simulink model "Baterie"  (R2023b)
settings: Solver=FixedStepAuto  StartTime=0.0  StopTime=10000  FixedStep=0.01  RelTol=1e-3
undefined symbols (not defined in the file): Cp_sys, Cp_sys1, Cp_sys2, Rp_sys, Rp_sys1, Rp_sys2, Rs_sys
libraries: simulink x1
settings Model: Creator=tudorn  LastModifiedBy=tudorn

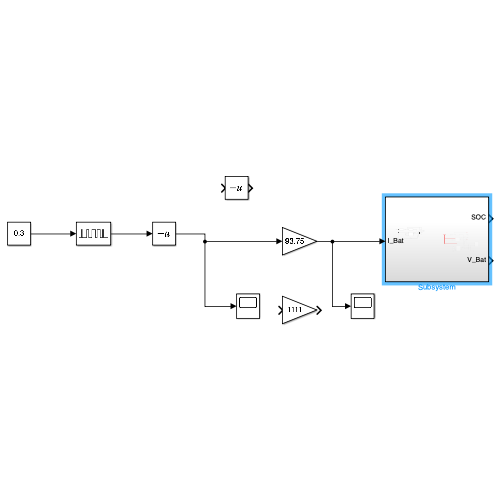
[thumbnail: Simulink's stored preview of the top-level diagram]
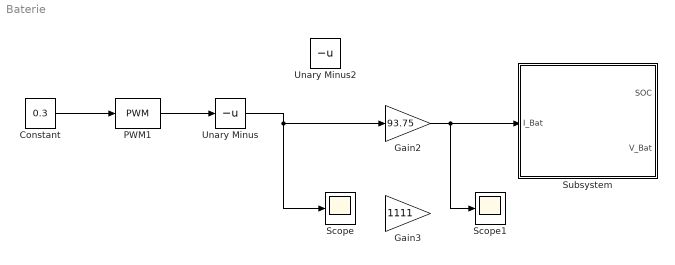
== system Baterie ==
  Constant : Constant  Value=0.3
  Gain2 : Gain  Gain=93.75
  Gain3 : Gain  Gain=1111
  PWM1 : simulink/Discontinuities/PWM  DisableCoverage=on  Period=1000  InitialDelay=0  DisallowZeroDutyCycle=off  RunAtFixedTimeIntervals=on  SampleTime=0.01
  Scope : Scope
  Scope1 : Scope
  Subsystem : Subsystem
  Unary Minus : UnaryMinus
  Unary Minus2 : UnaryMinus
  wires:
  Constant/1 -> PWM1/1
  Gain2/1 -> Scope1/1, Subsystem/1(I_Bat)
  PWM1/1 -> Unary Minus/1
  Unary Minus/1 -> Gain2/1, Scope/1

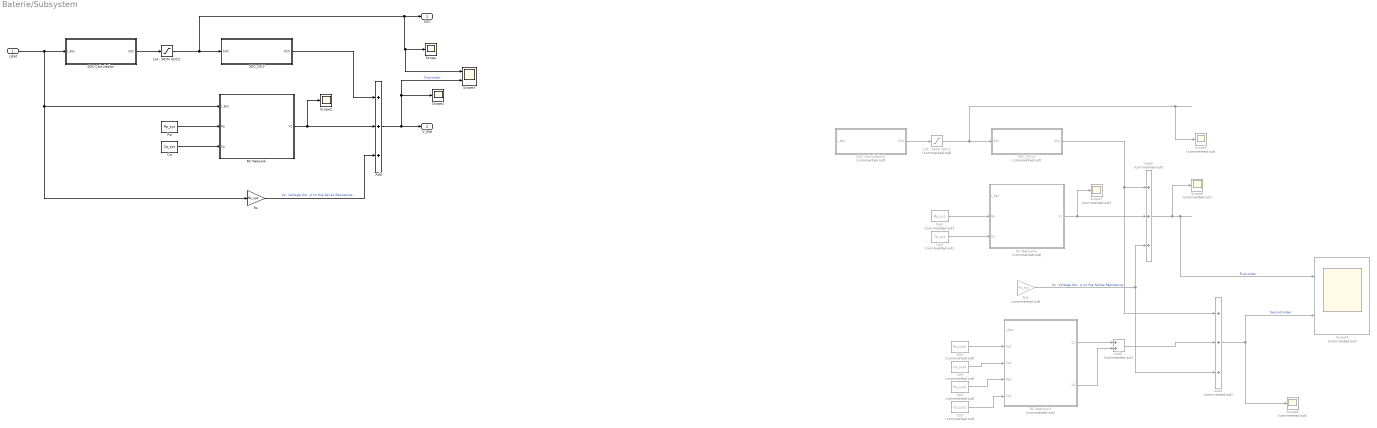
== system Baterie/Subsystem ==
  I_Bat : Inport
  (14 - 96)% SOC1 : Saturate  Commented=on  UpperLimit=96  LowerLimit=14
  (14 - 96)% SOC2 : Saturate  UpperLimit=96  LowerLimit=14
  Add : Sum  Inputs=+++
  Add3 : Sum  Commented=on  Inputs=+++
  Add4 : Sum  Commented=on  Inputs=+++
  Add5 : Sum  Commented=on
  Cp : Constant  Value=Cp_sys
  Cp3 : Constant  Commented=on  Value=Cp_sys
  Cp4 : Constant  Commented=on  Value=Cp_sys1
  Cp5 : Constant  Commented=on  Value=Cp_sys2
  RC Network : Subsystem
  RC Network2 : Subsystem  Commented=on
  RC Network3 : Subsystem  Commented=on
  Rp : Constant  Value=Rp_sys
  Rp3 : Constant  Commented=on  Value=Rp_sys
  Rp4 : Constant  Commented=on  Value=Rp_sys1
  Rp5 : Constant  Commented=on  Value=Rp_sys2
  Rs : Gain  Gain=Rs_sys
  Rs1 : Gain  Commented=on  Gain=Rs_sys
  SOC Calculation : Subsystem
  SOC Calculation1 : Subsystem  Commented=on
  SOC_OCV : Subsystem
  SOC_OCV1 : Subsystem  Commented=on
  Scope : Scope
  Scope1 : Scope
  Scope2 : Scope
  Scope3 : Scope  NumInputPorts=2
  Scope{5..8} (4 alike) : Scope  Commented=on
  Scope9 : Scope  Commented=on  NumInputPorts=2
  SOC : Outport
  V_Bat : Outport  Port=2
  wires:
  RC Network/1(V1) -> Scope2/1, Add/2
  SOC_OCV/1(OCV) -> Add/1
  Rp/1 -> RC Network/2(Rp)
  Cp/1 -> RC Network/3(Cp)
  I_Bat/1 -> SOC Calculation/1(I_Bat), Rs/1, RC Network/1(I_Bat)
  Add/1 -> Scope3/2, Scope1/1, V_Bat/1  "First-order"
  Rs/1 -> Add/3  "Vs - Voltage drop on the Series Resistance"
  Add4/1 -> Scope9/2, Scope8/1  "Second order"
  Add5/1 -> Add4/2
  RC Network3/2(V2) -> Add5/2
  RC Network3/1(V1) -> Add5/1
  Cp5/1 -> RC Network3/5(Cp2)
  Rp5/1 -> RC Network3/4(Rp2)
  Rp4/1 -> RC Network3/2(Rp1)
  Cp4/1 -> RC Network3/3(Cp1)
  (14 - 96)% SOC1/1 -> SOC_OCV1/1(SOC), Scope5/1
  Rs1/1 -> Add3/3, Add4/3  "Vs - Voltage drop on the Series Resistance"
  SOC Calculation1/1(SOC) -> (14 - 96)% SOC1/1
  Add3/1 -> Scope9/1, Scope6/1  "First-order"
  ? -> RC Network2/1(I_Bat), Rs1/1, RC Network3/1(I_Bat), SOC Calculation1/1(I_Bat)
  Cp3/1 -> RC Network2/3(Cp)
  Rp3/1 -> RC Network2/2(Rp)
  SOC_OCV1/1(OCV) -> Add3/1, Add4/1
  RC Network2/1(V1) -> Add3/2, Scope7/1
  SOC Calculation/1(SOC) -> (14 - 96)% SOC2/1
  (14 - 96)% SOC2/1 -> Scope3/1, Scope/1, SOC/1, SOC_OCV/1(SOC)

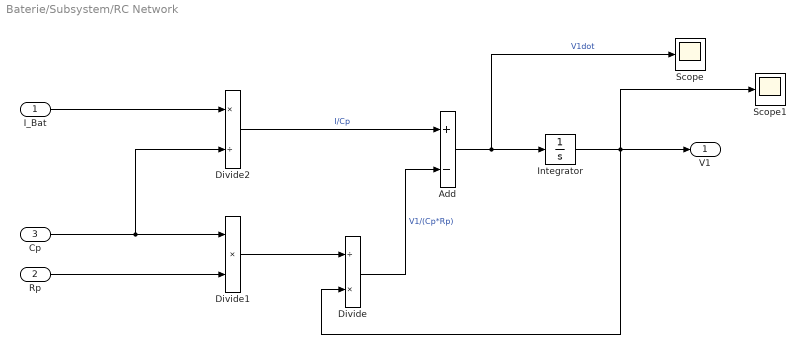
== system Baterie/Subsystem/RC Network ==
  I_Bat : Inport
  Rp : Inport  Port=2
  Cp : Inport  Port=3
  Add : Sum  Inputs=+-
  Divide : Product  Inputs=/*
  Divide1 : Product  Inputs=**
  Divide2 : Product  Inputs=*/
  Integrator : Integrator
  Scope : Scope
  Scope1 : Scope
  V1 : Outport
  wires:
  Cp/1 -> Divide2/2, Divide1/1
  Rp/1 -> Divide1/2
  I_Bat/1 -> Divide2/1
  Divide2/1 -> Add/1  "I/Cp"
  Add/1 -> Scope/1, Integrator/1  "V1dot"
  Divide/1 -> Add/2  "V1/(Cp*Rp)"
  Divide1/1 -> Divide/1
  Integrator/1 -> Scope1/1, V1/1, Divide/2

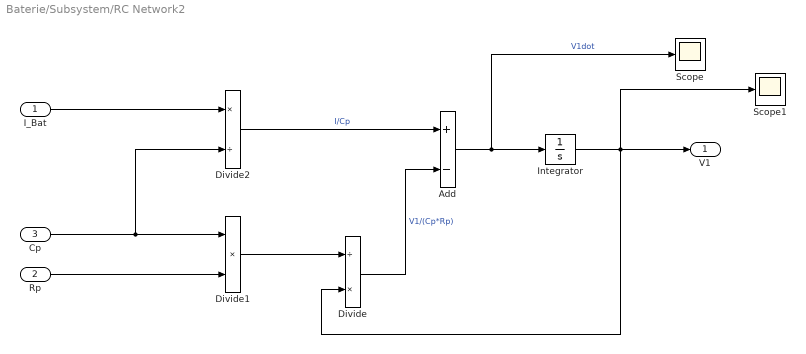
== system Baterie/Subsystem/RC Network2 ==
  I_Bat : Inport
  Rp : Inport  Port=2
  Cp : Inport  Port=3
  Add : Sum  Inputs=+-
  Divide : Product  Inputs=/*
  Divide1 : Product  Inputs=**
  Divide2 : Product  Inputs=*/
  Integrator : Integrator
  Scope : Scope
  Scope1 : Scope
  V1 : Outport
  wires:
  Integrator/1 -> Divide/2, V1/1, Scope1/1
  Divide1/1 -> Divide/1
  Divide/1 -> Add/2  "V1/(Cp*Rp)"
  Add/1 -> Integrator/1, Scope/1  "V1dot"
  Divide2/1 -> Add/1  "I/Cp"
  I_Bat/1 -> Divide2/1
  Rp/1 -> Divide1/2
  Cp/1 -> Divide1/1, Divide2/2

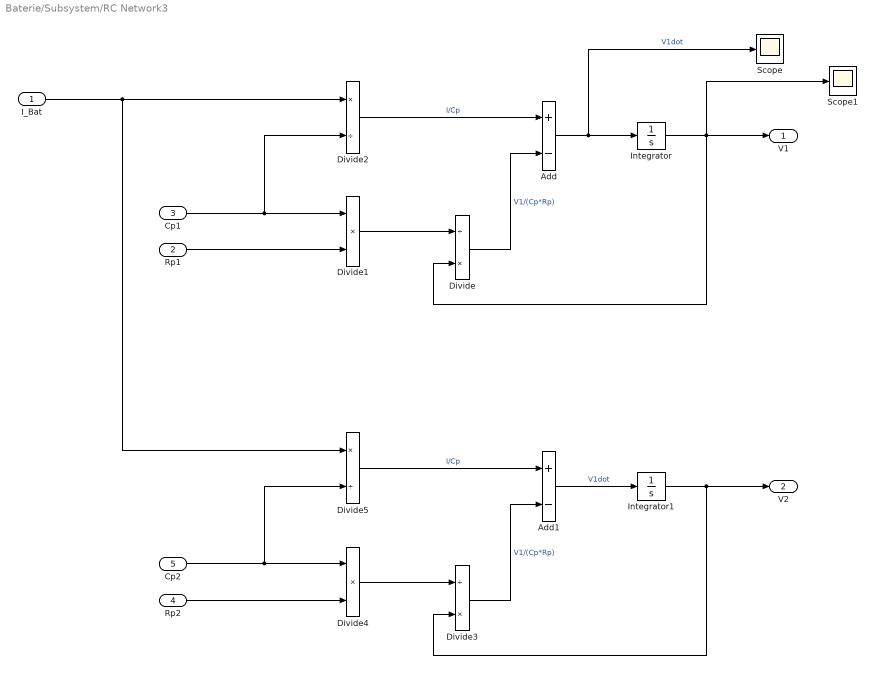
== system Baterie/Subsystem/RC Network3 ==
  I_Bat : Inport
  Rp1 : Inport  Port=2
  Cp1 : Inport  Port=3
  Rp2 : Inport  Port=4
  Cp2 : Inport  Port=5
  Add : Sum  Inputs=+-
  Add1 : Sum  Inputs=+-
  Divide : Product  Inputs=/*
  Divide1 : Product  Inputs=**
  Divide2 : Product  Inputs=*/
  Divide3 : Product  Inputs=/*
  Divide4 : Product  Inputs=**
  Divide5 : Product  Inputs=*/
  Integrator : Integrator
  Integrator1 : Integrator
  Scope : Scope
  Scope1 : Scope
  V1 : Outport
  V2 : Outport  Port=2
  wires:
  Divide5/1 -> Add1/1  "I/Cp"
  Rp2/1 -> Divide4/2
  Cp2/1 -> Divide4/1, Divide5/2
  Divide3/1 -> Add1/2  "V1/(Cp*Rp)"
  Divide4/1 -> Divide3/1
  Integrator1/1 -> Divide3/2, V2/1
  Add1/1 -> Integrator1/1  "V1dot"
  Integrator/1 -> Divide/2, V1/1, Scope1/1
  Divide1/1 -> Divide/1
  Divide/1 -> Add/2  "V1/(Cp*Rp)"
  Add/1 -> Integrator/1, Scope/1  "V1dot"
  Divide2/1 -> Add/1  "I/Cp"
  I_Bat/1 -> Divide2/1, Divide5/1
  Rp1/1 -> Divide1/2
  Cp1/1 -> Divide1/1, Divide2/2

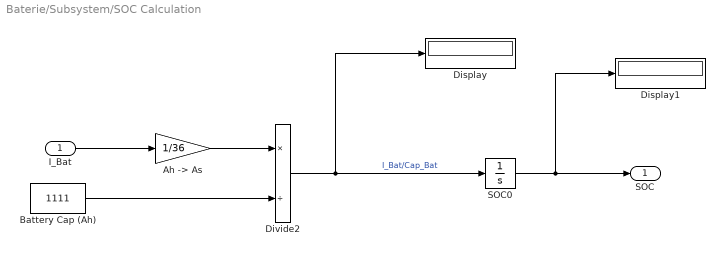
== system Baterie/Subsystem/SOC Calculation ==
  I_Bat : Inport
  "Ah -> As" : Gain  Gain=1/36
  Battery Cap (Ah) : Constant  Value=1111
  Display : Display
  Display1 : Display
  Divide2 : Product  Inputs=*/
  SOC0 : Integrator  InitialCondition=75
  SOC : Outport
  wires:
  SOC0/1 -> Display1/1, SOC/1
  Divide2/1 -> Display/1, SOC0/1  "I_Bat/Cap_Bat"
  I_Bat/1 -> "Ah -> As"/1
  Battery Cap (Ah)/1 -> Divide2/2
  "Ah -> As"/1 -> Divide2/1

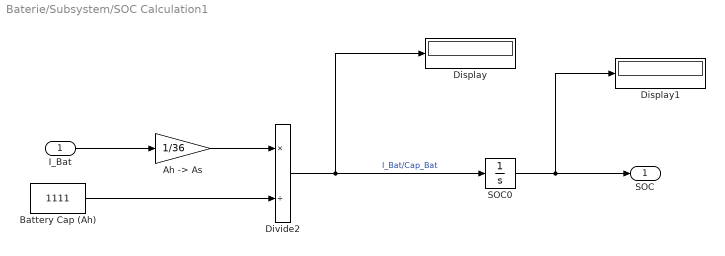
== system Baterie/Subsystem/SOC Calculation1 ==
  I_Bat : Inport
  "Ah -> As" : Gain  Gain=1/36
  Battery Cap (Ah) : Constant  Value=1111
  Display : Display
  Display1 : Display
  Divide2 : Product  Inputs=*/
  SOC0 : Integrator  InitialCondition=75
  SOC : Outport
  wires:
  "Ah -> As"/1 -> Divide2/1
  Battery Cap (Ah)/1 -> Divide2/2
  I_Bat/1 -> "Ah -> As"/1
  Divide2/1 -> SOC0/1, Display/1  "I_Bat/Cap_Bat"
  SOC0/1 -> SOC/1, Display1/1

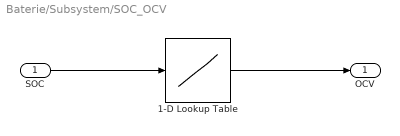
== system Baterie/Subsystem/SOC_OCV ==
  SOC : Inport
  1-D Lookup Table : Lookup_n-D  NumberOfTableDimensions=1  BreakpointsForDimension1=[0 5 9.5 14 20 30 40 50 60 70 80 90 96 99 99.5 100]  Table=[40, 44.8, 48, 50.40, 51.20, 51.60, 52, 52.20, 52.40, 52.80, 53.20, 53.60, 52.80, 54, 55.20, 58.40]  InternalRulePriority=Speed  RndMeth=Simplest
  OCV : Outport
  wires:
  SOC/1 -> 1-D Lookup Table/1
  1-D Lookup Table/1 -> OCV/1

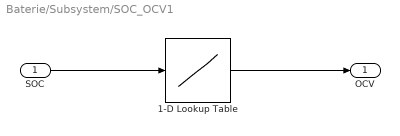
== system Baterie/Subsystem/SOC_OCV1 ==
  SOC : Inport
  1-D Lookup Table : Lookup_n-D  NumberOfTableDimensions=1  BreakpointsForDimension1=[0 5 9.5 14 20 30 40 50 60 70 80 90 96 99 99.5 100]  Table=[40, 44.8, 48, 50.40, 51.20, 51.60, 52, 52.20, 52.40, 52.80, 53.20, 53.60, 52.80, 54, 55.20, 58.40]  InternalRulePriority=Speed  RndMeth=Simplest
  OCV : Outport
  wires:
  1-D Lookup Table/1 -> OCV/1
  SOC/1 -> 1-D Lookup Table/1
